simulink library "tvb"  (Simulink 8.1)
settings: Solver=ode1  StartTime=0.0  StopTime=Inf  FixedStep=0.001  RelTol=1e-3
PostLoadFcn:
  | , if any(exist('dsrtsu_mdlpostloadfcn', 'file') == [2, 3, 6]), try dsrtsu_mdlpostloadfcn('Execute', bdroot); catch fprintf('Error in PostLoadFcn (dsrtsu_mdlpostloadfcn) for model "%s":\n %s\n', bdroot, lasterr); end, end,
undefined symbols (not defined in the file or in its folder): KACC_ACCDistCtrlTargetDecelThres_mps2, KACC_ACCTargetDecelOffThres_mps2, KACC_ACCTargetDecelThres_mps2
libraries: hcu_lib x1, tvd x1
settings Model: DSRTSU_INTERNAL_RTI_VER=450  DSRTSU_INTERNAL_RTI_TYPE=rti1401  RTICANMMDATA=struct('GeneralSetupData',struct('modelroot','D:\ELN150201_TAIWAN\trunk\AdasDragon\software\sw_development\arch\app\acc','generalsettings',struct('filesettings',struct('destfolder',struct('Name','RTICANMM_FILES','Check',1),'buildfolder',struct('Name','.','Check',1),'AbsDestfolder',struct('Name','D:\ELN150201_TAIWAN\trunk\AdasDragon\software\sw_development\arch\app\acc\RTICANMM_FILES'),'AbsBuildfolder',struct('Name','D:\ELN150201_TAIWAN\trunk\AdasDragon\software\sw_development\arch\app\acc'))),'options',struct('addpaths',1,'rmpaths',1,'addtrcexclusion',logical(1),'cannavigator',struct('checkmonitoring',0),'show_usrtrc',0,'use_usrtrc',0),'advanced',struct('options',[1 1 1 1 1 1 1 1 1 1 1 1 1 1 1 1 1 1 1 1 1 1 1 1 1 1 1 1 1 1 1 1 1 1 1 1 1 1 1 1 1 1 1 1 1 1 1 1 1 1 1 1 1 1 1 1 1 1 1 1 1 1 1 1 1 1 1 1 1 1 1 1 1 1 1 1 1 1 1 1 1 1 1 1 1 1 1 1 1 1 1 1 1 1 1 1 1 1 1 1]),'MPSetup',{{}},'modelname','tvb','block','tvb'))  DSRTSU_INTERNAL_RTIFPGA=40  Creator=AT015411  LastModifiedBy=AT015555

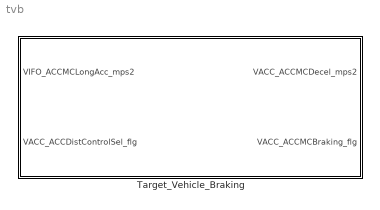
== system tvb ==
  Target_Vehicle_Braking : Subsystem

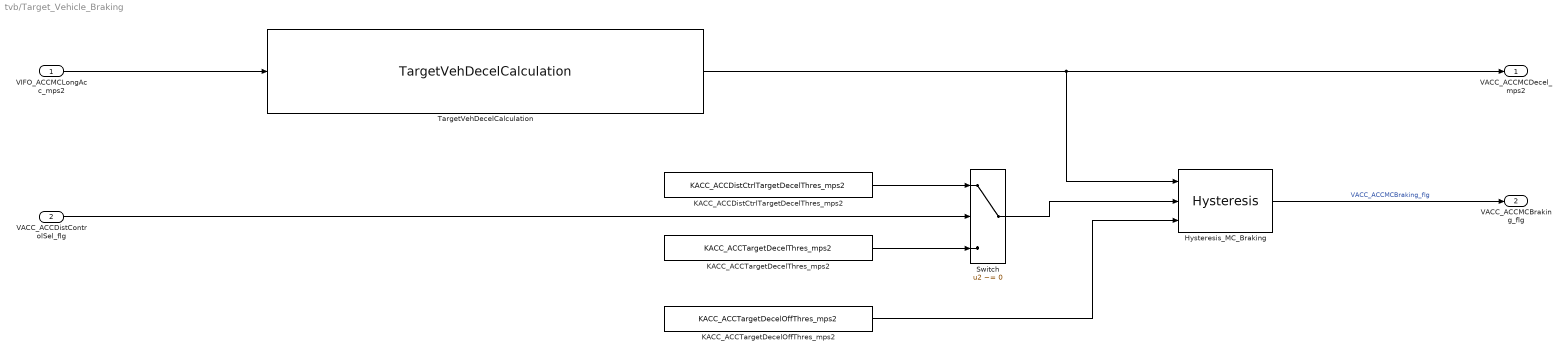
== system tvb/Target_Vehicle_Braking ==
  VIFO_ACCMCLongAcc_mps2 : Inport
  VACC_ACCDistControlSel_flg : Inport  Port=2
  Hysteresis_MC_Braking : hcu_lib/Hysteresis  SystemSampleTime=-1
  KACC_ACCDistCtrlTargetDecelThres_mps2 : Constant  Value=KACC_ACCDistCtrlTargetDecelThres_mps2
  KACC_ACCTargetDecelOffThres_mps2 : Constant  Value=KACC_ACCTargetDecelOffThres_mps2
  KACC_ACCTargetDecelThres_mps2 : Constant  Value=KACC_ACCTargetDecelThres_mps2
  Switch : Switch  Criteria=u2 ~= 0
  TargetVehDecelCalculation : tvd/TargetVehDecelCalculation
  VACC_ACCMCDecel_mps2 : Outport
  VACC_ACCMCBraking_flg : Outport  Port=2
  wires:
  VACC_ACCDistControlSel_flg/1 -> Switch/2
  VIFO_ACCMCLongAcc_mps2/1 -> TargetVehDecelCalculation/1
  Hysteresis_MC_Braking/1 -> VACC_ACCMCBraking_flg/1  "VACC_ACCMCBraking_flg"
  TargetVehDecelCalculation/1 -> Hysteresis_MC_Braking/1, VACC_ACCMCDecel_mps2/1
  KACC_ACCTargetDecelThres_mps2/1 -> Switch/3
  KACC_ACCDistCtrlTargetDecelThres_mps2/1 -> Switch/1
  Switch/1 -> Hysteresis_MC_Braking/2
  KACC_ACCTargetDecelOffThres_mps2/1 -> Hysteresis_MC_Braking/3
